simulink model "SpringMass_Model_TDomain"  (R2020a)
settings: Solver=VariableStepAuto  StartTime=0.0  StopTime=10  MaxStep=0.05  RelTol=1e-3
values from neighbouring files (symbols this model uses):
  b = 1.8    [SpringMass_mScript_SDomain.m]    (also in SpringMass_mScript_TDomain.m = 2)
  F = 10    [SpringMass_mScript_SDomain.m]    (also in SpringMass_mScript_TDomain.m)
  k = 10    [SpringMass_mScript_SDomain.m]    (also in SpringMass_mScript_TDomain.m = 20)
  M = 1    [SpringMass_mScript_SDomain.m]    (also in SpringMass_mScript_TDomain.m)
settings Model: Creator=alexd  LastModifiedBy=alexd

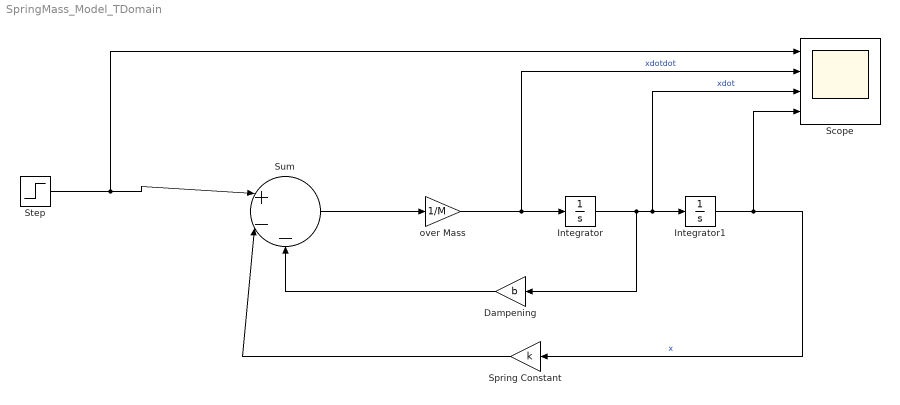
== system SpringMass_Model_TDomain ==
  Dampening : Gain  Gain=b
  Integrator : Integrator
  Integrator1 : Integrator
  Scope : Scope  NumInputPorts=4
  Spring Constant : Gain  Gain=k
  Step : Step  After=F  SampleTime=0
  Sum : Sum  Inputs=|+--
  over Mass : Gain  Gain=1/M
  wires:
  over Mass/1 -> Scope/2, Integrator/1  "xdotdot"
  Integrator/1 -> Dampening/1, Scope/3, Integrator1/1  "xdot"
  Integrator1/1 -> Scope/4, Spring Constant/1  "x"
  Dampening/1 -> Sum/3
  Spring Constant/1 -> Sum/2
  Sum/1 -> over Mass/1
  Step/1 -> Scope/1, Sum/1
